simulink model "PEM_AFC"  (R2024a)
settings: Solver=FixedStepDiscrete  StartTime=0.0  StopTime=60  RelTol=1e-3  EnableMultiTasking=on
values from neighbouring files (symbols this model uses):
  alpha_bab = sqrt(Es / (SNR_linear * En_bab))    [Init_noise.m]
  alpha_imp = sqrt(Es / (SIR_linear * En_imp))    [Init_noise.m]
undefined symbols (not defined in the file or in its folder): a, delta, dfilt, dg, dk, framelength, g2, g4, mug, n_imp
libraries: dspobslib x6, dspvision x2, dspsrcs4 x2, dspswit3 x1, dspbuff3 x1, dspstat3 x1, dspsolvers x1, dspmathops x1
settings Model: Creator=Renato_Nakagawa  LastModifiedBy=tienc
settings SolverCC: AlgebraicLoopSolver=TrustRegion
settings DataIOCC: LimitDataPoints=on  SaveFormat=Array  ReturnWorkspaceOutputs=off
settings OptimizationCC: DefaultParameterBehavior=Inlined  EnhancedBackFolding=on  PassReuseOutputArgsAs=Individual arguments  ZeroExternalMemoryAtStartup=off  ZeroInternalMemoryAtStartup=off  OptimizeBlockOrder=speed  DifferentSizesBufferReuse=on  OptimizationCustomize=off  EfficientTunableParamExpr=on
settings DebuggingCC: UnderspecifiedInitializationDetection=Classic  MergeDetectMultiDrivingBlocksExec=none  SolverPrmCheckMsg=warning  ParameterTunabilityLossMsg=error  UnconnectedInputMsg=warning  UnconnectedOutputMsg=warning  UnconnectedLineMsg=warning  StateNameClashWarn=warning  SFUnexpectedBacktrackingDiag=warning  SFNoUnconditionalDefaultTransitionDiag=warning  SFExecutionAtInitializationDiag=none  ArithmeticOperatorsInVariantConditions=warning
settings HardwareCC: ProdBitPerPointer=32  ProdBitPerSizeT=32  ProdBitPerPtrDiffT=32  ProdLargestAtomicFloat=None  ProdIntDivRoundTo=Undefined  ProdEndianess=Unspecified  ProdWordSize=32  ProdHWDeviceType=32-bit Generic
settings ModelReferenceCC: PropagateSignalLabelsOutOfModel=off
settings SFSimCC: SimUseLocalCustomCode=off  MATLABDynamicMemAlloc=off  CustomCodeUndefinedFunction=UseInterfaceOnly
settings RTWCC: Description=Embedded Coder  SystemTargetFile=ert.tlc  GenCodeOnly=on  TemplateMakefile=ert_default_tmf  RTWUseLocalCustomCode=off  GPUComputeCapability=3.5
settings CodeAppCC: ForceParamTrailComments=on  IgnoreCustomStorageClasses=off  OperatorAnnotations=on  SimulinkDataObjDesc=on  SFDataObjDesc=on  InsertBlockDesc=on
settings ERTTargetCC: GenerateSampleERTMain=on  InlinedParameterPlacement=NonHierarchical  ERTCustomFileTemplate=example_file_process.tlc
settings ConfigComp: CovMetricSettings=dw  CovSaveCumulativeToWorkspaceVar=on  CovSaveSingleToWorkspaceVar=on  CovExternalEMLEnable=off  CovSFcnEnable=off

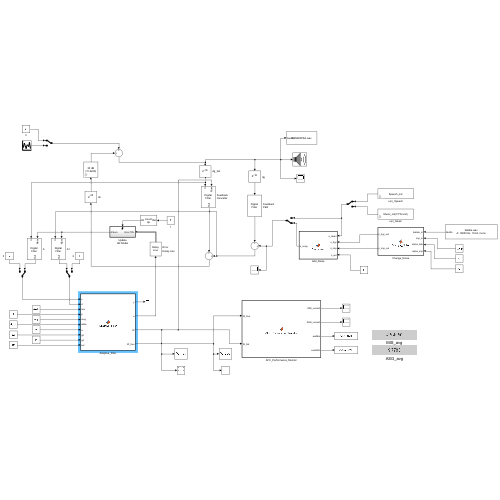
[thumbnail: Simulink's stored preview of the top-level diagram]
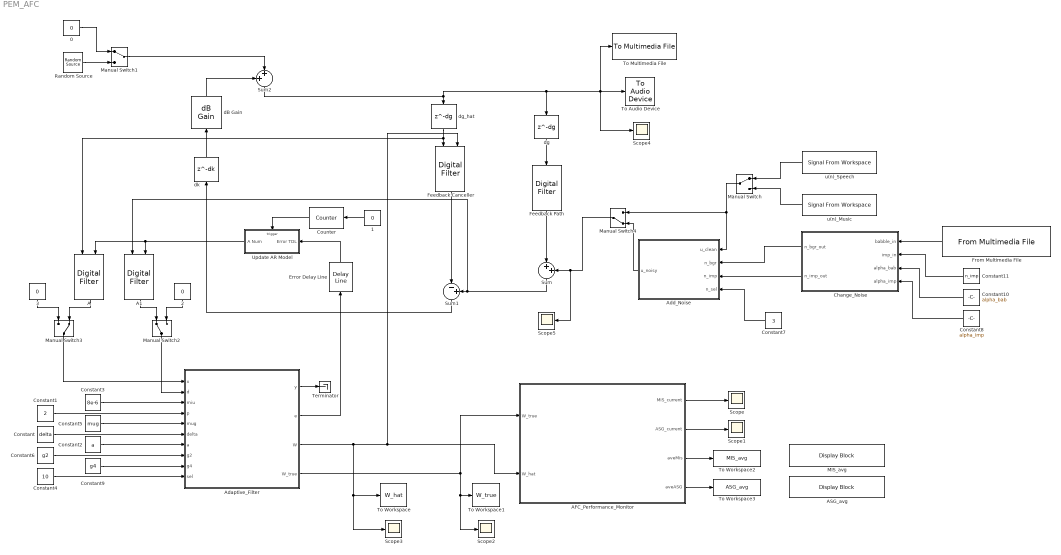
== system PEM_AFC ==
  {0..3} (4 alike) : Constant  Value=0
  A : dspobslib/Digital Filter  TypePopup=FIR (all zeros)  IIRFiltStruct=Direct form II transposed  AllPoleFiltStruct=Direct form  FIRFiltStruct=Direct form  CoeffSource=Input port(s)  NumCoeffs=g2  DenCoeffs=[1 0.1]  BiQuadCoeffs=[1 0.3 0.4 1 0.1 0.2]  LatticeCoeffs=[0.2 0.4]  denIgnore=on  FiltPerSampPopup=One filter per frame  IC=0  ICnum=0  ICden=0  roundingMode=Floor  overflowMode=off  ScaleValues=1  scaleValueFracLength=14  stageInFracLength=15  stageOutFracLength=15  FilterSource=Input port(s)  dfiltObjectName=dfilt.dffir([1 2 1])
  A1 : dspobslib/Digital Filter  TypePopup=FIR (all zeros)  IIRFiltStruct=Direct form II transposed  AllPoleFiltStruct=Direct form  FIRFiltStruct=Direct form  CoeffSource=Input port(s)  NumCoeffs=g2  DenCoeffs=[1 0.1]  BiQuadCoeffs=[1 0.3 0.4 1 0.1 0.2]  LatticeCoeffs=[0.2 0.4]  denIgnore=on  FiltPerSampPopup=One filter per frame  IC=0  ICnum=0  ICden=0  roundingMode=Floor  overflowMode=off  ScaleValues=1  scaleValueFracLength=14  stageInFracLength=15  stageOutFracLength=15  FilterSource=Input port(s)  dfiltObjectName=dfilt.dffir([1 2 1])
  AFC_Performance_Monitor : MATLAB Function  TreatAsAtomicUnit=on
  ASG_avg : DisplayBlock  LabelPosition=Hide  Transparency=1
  Adaptive_Filter : MATLAB Function  TreatAsAtomicUnit=on
  Add_Noise : MATLAB Function  TreatAsAtomicUnit=on
  Change_Noise : MATLAB Function  TreatAsAtomicUnit=on
  Constant : Constant  Value=delta
  Constant1 : Constant  Value=2
  Constant10 : Constant  Value=alpha_bab
  Constant11 : Constant  Value=n_imp
  Constant2 : Constant  Value=a
  Constant3 : Constant  Value=8e-6
  Constant4 : Constant  Value=10
  Constant5 : Constant  Value=mug
  Constant6 : Constant  Value=g2
  Constant7 : Constant  Value=3
  Constant8 : Constant  Value=alpha_imp
  Constant9 : Constant  Value=g4
  Counter : dspswit3/Counter  Direction=Up  CountEvent=Free running  CounterSize=User defined  MaxCount=framelength-1  InitialCount=0  Output=Hit  HitValue=framelength-1  ResetInput=on  SamplesPerFrame=1  Ts=1/16000  CntDtype=double  HitDtype=Boolean
  Error Delay Line : dspbuff3/Delay Line  siz=Nh  ic=0  directfeed=off  enable_output=off  hold_output=off  OutputFrames=on
  Feedback Canceller : dspobslib/Digital Filter  TypePopup=FIR (all zeros)  IIRFiltStruct=Direct form II transposed  AllPoleFiltStruct=Direct form  FIRFiltStruct=Direct form  CoeffSource=Input port(s)  NumCoeffs=g2  DenCoeffs=[1 0.1]  BiQuadCoeffs=[1 0.3 0.4 1 0.1 0.2]  LatticeCoeffs=[0.2 0.4]  denIgnore=on  FiltPerSampPopup=One filter per frame  IC=0  ICnum=0  ICden=0  roundingMode=Floor  overflowMode=off  ScaleValues=1  scaleValueFracLength=14  stageInFracLength=15  stageOutFracLength=15  FilterSource=Input port(s)  dfiltObjectName=dfilt.dffir([1 2 1])
  "Feedback Path " : dspobslib/Digital Filter  TypePopup=FIR (all zeros)  IIRFiltStruct=Direct form II transposed  AllPoleFiltStruct=Direct form  FIRFiltStruct=Direct form  CoeffSource=Specify via dialog  NumCoeffs=g2  DenCoeffs=[1 0.1]  BiQuadCoeffs=[1 0.3 0.4 1 0.1 0.2]  LatticeCoeffs=[0.2 0.4]  denIgnore=on  FiltPerSampPopup=One filter per frame  IC=0  ICnum=0  ICden=0  roundingMode=Floor  overflowMode=off  ScaleValues=1  scaleValueFracLength=14  stageInFracLength=15  stageOutFracLength=15  FilterSource=Specify via dialog  dfiltObjectName=dfilt.dffir([1 2 1])
  From Multimedia File : dspvision/From Multimedia File  inputFilename=C:\Documents\NCKH\IPAPSA for AFC using prefilter in HAs\Simulink\NOISEX-92\babble.wav  readRange=[1 Inf]  loop=on  numPlays=inf  outputStreams=Audio only  videoDataType=single  audioDataType=double  inheritSampleTime=off  userDefinedSampleTime=1/16000  noAudioOutput=off  isIntensityVideo=off  fourcc=RGB  colorVideoFormat=Separate color signals  outputEOF=off  dataOrg=Column-major  audioFrameSize=1  computeAudioFrameSize=off  outSamplingMode=Sample based
      settings: LibrarySourceBlock=audiosources/From Multimedia File
  MIS_avg : DisplayBlock  LabelPosition=Hide  Transparency=1
  Manual Switch : ManualSwitch
  Manual Switch1 : ManualSwitch
  Manual Switch2 : ManualSwitch
  Manual Switch3 : ManualSwitch  CurrentSetting=0
  Manual Switch4 : ManualSwitch  CurrentSetting=0
  Random Source : dspobslib/Random Source  SrcType=Gaussian  NormMethod=Ziggurat  CltLength=12  MinVal=0  MaxVal=1  MeanVal=0  VarVal=var  RepMode=Not repeatable  rawSeed=1  IsInherit=off  SampMode=Discrete  SampTime=1/16000  SampFrame=1  DataType=Double  OutComplex=Real  OutputFrames=on
  Scope{,1..5} (6 alike) : Scope
  Sum : Sum  Inputs=|++
  Sum1 : Sum  Inputs=|-+
  Sum2 : Sum  Inputs=++|
  Terminator : Terminator
  To Audio Device : dspobslib/To Audio Device  deviceName=Default  inheritSampleRate=on  sampleRate=44100  deviceDatatype=Determine from input data type  autoBufferSize=on  bufferSize=4096  queueDuration=1.0  defaultOutputChannelMapping=on  outputChannelMapping=1  outputNumUnderrunSamples=off
  To Multimedia File : dspvision/To Multimedia File  outputFilename=BSMIPAPSA.wav  streamSelection=Audio only  videoCompressor=None (uncompressed)  audioCompressor=None (uncompressed)  imagePorts=One multidimensional signal  fileType=WAV  audioDatatype=16-bit integer  fourcc=RGB  audioBitRate=128  audioQuality=75  videoQuality=75  mj2000CompFactor=10
      settings: LibrarySourceBlock=audiosinks/To Multimedia File
  To Workspace : ToWorkspace  VariableName=W_hat  SampleTime=-1
      settings: Save2DSignal=2-D array (concatenate along first dimension)
  To Workspace1 : ToWorkspace  VariableName=W_true  SampleTime=-1
      settings: Save2DSignal=2-D array (concatenate along first dimension)
  To Workspace2 : ToWorkspace  VariableName=MIS_avg  SampleTime=-1
      settings: Save2DSignal=2-D array (concatenate along first dimension)
  To Workspace3 : ToWorkspace  VariableName=ASG_avg  SampleTime=-1
      settings: Save2DSignal=2-D array (concatenate along first dimension)
  Update AR Model : Subsystem  TreatAsAtomicUnit=on
  dB Gain : dspmathops/dB Gain  dB=K_dB  intype=Amplitude
  dg : Delay  DelayLength=dg  InitialCondition=0
  dg_hat : Delay  DelayLength=dg  InitialCondition=0
  dk : Delay  DelayLength=dk  InitialCondition=0
  u(n)_Music : dspsrcs4/Signal From Workspace  X=Music_m4(15*fs:end)  Ts=1/16000  nsamps=1  OutputAfterFinalValue=Setting to zero  ignoreOrWarnInputAndFrameLengths=off  OutputFrames=on
  u(n)_Speech : dspsrcs4/Signal From Workspace  X=Speech_m2  Ts=1/16000  nsamps=1  OutputAfterFinalValue=Setting to zero  ignoreOrWarnInputAndFrameLengths=off  OutputFrames=on
  wires:
  dk/1 -> dB Gain/1
  dg_hat/1 -> Feedback Canceller/1, A/1
  Sum1/1 -> dk/1
  dB Gain/1 -> Sum2/1
  Error Delay Line/1 -> Update AR Model/1(Error TDL)
  Counter/1 -> Update AR Model/Trigger
  Sum/1 -> Sum1/2, A1/1
  Update AR Model/1(A Num) -> A1/2, A/2
  u(n)_Speech/1 -> Manual Switch/1
  u(n)_Music/1 -> Manual Switch/2
  Manual Switch1/1 -> Sum2/2
  Random Source/1 -> Manual Switch1/2
  0/1 -> Manual Switch1/1
  1/1 -> Counter/1
  Constant5/1 -> Adaptive_Filter/5(mug)
  Adaptive_Filter/1(y) -> Terminator/1
  Adaptive_Filter/2(e) -> Error Delay Line/1
  Constant/1 -> Adaptive_Filter/6(delta)
  Constant1/1 -> Adaptive_Filter/4(p)
  Constant2/1 -> Adaptive_Filter/7(a)
  Constant4/1 -> Adaptive_Filter/10(sel)
  Constant3/1 -> Adaptive_Filter/3(miu)
  3/1 -> Manual Switch3/1
  A/1 -> Manual Switch3/2
  A1/1 -> Manual Switch2/1
  2/1 -> Manual Switch2/2
  Manual Switch3/1 -> Adaptive_Filter/1(x)
  Manual Switch2/1 -> Adaptive_Filter/2(d)
  AFC_Performance_Monitor/1(MIS_current) -> Scope/1
  Adaptive_Filter/3(W) -> Feedback Canceller/2, AFC_Performance_Monitor/2(W_hat), To Workspace/1, Scope3/1
  Sum2/1 -> To Multimedia File/1, Scope4/1, To Audio Device/1, dg/1, dg_hat/1
  Feedback Canceller/1 -> Sum1/1
  AFC_Performance_Monitor/3(aveMis) -> To Workspace2/1
  AFC_Performance_Monitor/4(aveASG) -> To Workspace3/1
  AFC_Performance_Monitor/2(ASG_current) -> Scope1/1
  dg/1 -> "Feedback Path "/1
  "Feedback Path "/1 -> Sum/1
  Constant6/1 -> Adaptive_Filter/8(g2)
  Constant9/1 -> Adaptive_Filter/9(g4)
  Adaptive_Filter/4(W_true) -> AFC_Performance_Monitor/1(W_true), Scope2/1, To Workspace1/1
  Constant7/1 -> Add_Noise/4(n_sel)
  Manual Switch/1 -> Manual Switch4/1, Add_Noise/1(u_clean)
  From Multimedia File/1 -> Change_Noise/1(babble_in)
  Constant10/1 -> Change_Noise/3(alpha_bab)
  Constant8/1 -> Change_Noise/4(alpha_imp)
  Change_Noise/1(n_bgr_out) -> Add_Noise/2(n_bgr)
  Change_Noise/2(n_imp_out) -> Add_Noise/3(n_imp)
  Constant11/1 -> Change_Noise/2(imp_in)
  Manual Switch4/1 -> Scope5/1, Sum/2
  Add_Noise/1(u_noisy) -> Manual Switch4/2

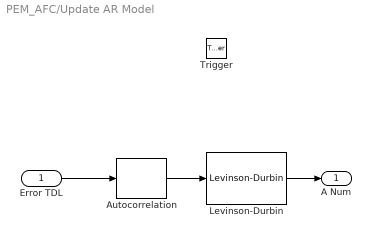
== system PEM_AFC/Update AR Model ==
  Error TDL : Inport
  Trigger : TriggerPort  VariantControl=(inherit)  ZeroCross=off
  Autocorrelation : dspstat3/Autocorrelation  AllPositiveLags=on  maxlag=1  bias=Unbiased  domain=Time  roundingMode=Floor  overflowMode=off  outputDataTypeStr=Inherit: Same as accumulator  outputMin=[]  outputMax=[]  outputLastDataTypeStr=Inherit: Same as accumulator
  Levinson-Durbin : dspsolvers/Levinson-Durbin  coeffOutFcn=OBSOLETE  coeffOutFcnActive=A  outP=off  zeroInpHandling=on  roundingMode=Floor  overflowMode=off  prodOutputMode=User-defined  prodOutputWordLength=32  prodOutputFracLength=30  prodOutputDataTypeStr=fixdt(1,32,30)  prodOutputLastDataTypeStr=fixdt(1,32,30)  accumMode=User-defined  accumWordLength=32  accumFracLength=30  accumDataTypeStr=fixdt(1,32,30)  accumLastDataTypeStr=fixdt(1,32,30)  firstCoeffMode=Binary point scaling  firstCoeffWordLength=16  firstCoeffFracLength=15  firstCoeffDataTypeStr=fixdt(1,16,15)  firstCoeffMin=[]  firstCoeffMax=[]  firstCoeffLastDataTypeStr=fixdt(1,16,15)  secondCoeffMode=Binary point scaling  secondCoeffWordLength=16  secondCoeffFracLength=15  secondCoeffDataTypeStr=fixdt(1,16,15)  secondCoeffMin=[]  secondCoeffMax=[]  secondCoeffLastDataTypeStr=fixdt(1,16,15)  outputMin=[]  outputMax=[]
      settings: allowOverrides=off
  A Num : Outport
  wires:
  Autocorrelation/1 -> Levinson-Durbin/1
  Error TDL/1 -> Autocorrelation/1
  Levinson-Durbin/1 -> A Num/1

== matlab function PEM_AFC/AFC_Performance_Monitor ==
  data: W_true input; W_hat input; MIS_current output; ASG_current output; aveMis output; aveASG output
function [MIS_current, ASG_current, aveMis, aveASG] = AFC_Performance_Monitor(W_true, W_hat)
% AFC_Performance_Monitor
% Tính MIS (Misalignment) và ASG (Added Stable Gain) theo từng mẫu để
% xuất trực tiếp sang Scope trong Simulink. Đồng thời duy trì giá trị
% trung bình (running average) của MIS và ASG trong suốt phiên mô phỏng.
%
% INPUTS:
%   W_true : vector hệ số feedback path thật (kích thước Lx1 hoặc 1xL)
%   W_hat  : vector hệ số ước lượng (kích thước Lx1 hoặc 1xL)
%
% OUTPUTS:
%   MIS_current : giá trị MIS hiện thời (dB)
%   ASG_current : giá trị ASG hiện thời (dB)
%   aveMis      : trung bình MIS tính đến thời điểm hiện tại (dB)
%   aveASG      : trung bình ASG tính đến thời điểm hiện tại (dB)

% Chuẩn hóa kích thước vector cột
g_current = W_true(:);
g_hat_current = W_hat(:);

% Độ dài bộ lọc và Nfreq đồng bộ theo MIS_cal.m / PEM_TDfeedback_Modified_simulink.m
filter_length = length(g_current);
if filter_length == 0
    MIS_current = 0; ASG_current = 0; aveMis = 0; aveASG = 0; return; %#ok<*NASGU>
end
Nfreq = filter_length;

% Biến persistent cho trung bình cộng dồn
persistent sumMIS sumASG nSamples
if isempty(nSamples)
    sumMIS = 0;
    sumASG = 0;
    nSamples = 0;
end

% Tiền xử lý đồng bộ MIS_cal.m / PEM_TDfeedback_Modified_simulink.m
% - Remove DC cho đường thật
% - Chèn trễ d_fb cho cả thật và ước lượng
d_fb = 16; % phải trùng với mô phỏng
g_true_nodc = g_current - mean(g_current);
g_true_delayed = [zeros(d_fb,1); g_true_nodc; 0];
g_hat_delayed  = [zeros(d_fb,1); g_hat_current];

% Phổ tần số của hệ số thật và ước lượng
G_freq = fft(g_true_delayed, Nfreq);
G_hat_freq = fft(g_hat_delayed, Nfreq);

% Sai số ước lượng ở miền tần số (nửa dải tần)
half_idx = 1:ceil(Nfreq/2);
G_tilde = G_freq(half_idx) - G_hat_freq(half_idx);

% MIS hiện thời (đồng bộ công thức)
den_norm = norm(G_freq(half_idx));
% Thêm eps nhỏ để tránh NaN trong mô phỏng số mà không thay đổi định nghĩa
MIS_current = 20*log10(norm(G_tilde)/(den_norm + eps));

% MSG và ASG hiện thời (đồng bộ phạm vi tần số của ASG: 1:Nfreq/2+1)
G_tilde_abs = abs(G_tilde);
MSG_current = 20*log10(min(1./(G_tilde_abs + eps)));
G_freq_abs = abs(G_freq(1:(Nfreq/2+1)));
ASG_current = MSG_current - 20*log10(min(1./(G_freq_abs + eps)));

% Cập nhật trung bình cộng dồn
nSamples = nSamples + 1;
sumMIS = sumMIS + MIS_current;
sumASG = sumASG + ASG_current;
aveMis = sumMIS / nSamples;
aveASG = sumASG / nSamples;

end

== matlab function PEM_AFC/Adaptive_Filter ==
  data: x input; d input; miu input; p input; y output; mug input; e output; W output; delta input; a input; g2 input; g4 input; sel input; W_true output
function [y, e, W, W_true] = Adaptive_Filter(x, d, miu, p, mug, delta, a, g2, g4, sel)
    % --- KHAI BÁO HẰNG SỐ CỐ ĐỊNH ---
    FILTER_ORDER = 64;   
    MAX_P = 10;
    AR_ORDER = 20;
    FRAMELENGTH = 160;
    
    % --- KIỂM TRA ĐẦU VÀO ---
    assert(p <= MAX_P);          
    assert(p >= 1);
    
    % Khởi tạo outputs
    y = 0.0;
    e = 0.0;
    W = zeros(FILTER_ORDER, 1);
    W_true = zeros(FILTER_ORDER, 1);

    % Persistent variables
    persistent AF AR;
    persistent sample_counter feedback_path_changed;
    persistent change_sample current_feedback_path;

    %% --- KHỞI TẠO (INITIALIZATION) ---
    if isempty(AF)
        % Khởi tạo AF structure
        AF.gTD = zeros(FILTER_ORDER, 1);
        AF.N = FILTER_ORDER;
        AF.mu = miu;
        AF.delta = delta;
        AF.TDLLs = zeros(FILTER_ORDER, 1);
        AF.TDLLswh = zeros(FILTER_ORDER, 1);
        
        % Khởi tạo mảng cho APA (Kích thước tĩnh MAX_P)
        AF.P = p; 
        AF.TDLLswh_d = zeros(FILTER_ORDER + MAX_P - 1, 1); 
        AF.TDLMicwh = zeros(MAX_P, 1);     
        AF.Lswh_ap = zeros(FILTER_ORDER, MAX_P); 
        
        AF.delta_IPAPA = 0;
        AF.mu1 = 0.5 * mug;
        AF.mu2 = 0.1 * mug;
        
        % Khởi tạo cho PEM-IPAPSA / PEM-MIPAPSA / PEM-BSMIPAPSA
        AF.Q_tilde_prev = zeros(FILTER_ORDER, MAX_P - 1);
        
        % Khởi tạo AR structure
        AR.N = AR_ORDER;
        AR.w = [1; zeros(AR_ORDER-1, 1)];
        AR.framelength = FRAMELENGTH;
        AR.frameindex = 0;
        AR.TDLMicdelay = zeros(FRAMELENGTH+1, 1);
        AR.TDLLsdelay = zeros(FRAMELENGTH+1, 1);
        % Đây là biến gây lỗi lúc nãy, nó đã được khai báo ở đây là TDLMicwh
        AR.TDLMicwh = zeros(AR_ORDER, 1); 
        AR.TDLLswh = zeros(AR_ORDER, 1);
        AR.frame = zeros(FRAMELENGTH, 1);
        
        % Feedback path logic
        sample_counter = 0;
        feedback_path_changed = false;
        change_sample = 480000;
        current_feedback_path = 1;
    end

    %% --- XỬ LÝ CHÍNH (MAIN PROCESSING) ---
    % Chuẩn hóa input
    if ~isscalar(x), x = x(1); end
    if ~isscalar(d), d = d(1); end

    % Feedback path switching
    sample_counter = sample_counter + 1;
    if sample_counter >= 960000
        sample_counter = 0;
        feedback_path_changed = false;
        current_feedback_path = 1;
    end
    if sample_counter >= change_sample && ~feedback_path_changed
        feedback_path_changed = true;
        current_feedback_path = 2;
    end

    AF.mu = miu;
    
    % 1. Cập nhật TDLLs
    AF.TDLLs = [x; AF.TDLLs(1:end-1,1)];
    
    % 2. Tính error signal
    e = d - AF.gTD' * AF.TDLLs;
    
    % 3. Clipping
    e = 2*tanh(0.5*e);
    
    % 4, 5. Delay & Filter signals
    [Micdelay, AR.TDLMicdelay] = delay_sample_inline(d, AR.framelength, AR.TDLMicdelay);
    [Lsdelay, AR.TDLLsdelay] = delay_sample_inline(x, AR.framelength, AR.TDLLsdelay);
    
    % [ĐÃ SỬA LỖI TẠI ĐÂY] Dùng đúng tên biến AR.TDLMicwh
    [Micwh, AR.TDLMicwh] = filter_sample_inline(Micdelay, AR.w, AR.TDLMicwh);
    [Lswh, AR.TDLLswh] = filter_sample_inline(Lsdelay, AR.w, AR.TDLLswh);

    % 6. Update AR-model
    AR.frame(2:AR.framelength) = AR.frame(1:AR.framelength-1);
    AR.frame(1) = e;
    
    % Levinson Logic
    if and(AR.frameindex == AR.framelength-1, AR.N-1 > 0)
        R = zeros(AR.N, 1);
        for j = 1:AR.N
            frame_segment = AR.frame(j:end);
            pad_zeros = zeros(j-1, 1);
            vec_mult = [frame_segment; pad_zeros];
            R(j,1) = (AR.frame' * vec_mult) / AR.framelength;
        end
        [ar_coeffs, ~] = levinson(R, AR.N-1);
        AR.w(1:length(ar_coeffs)) = ar_coeffs';
        AR.w(length(ar_coeffs)+1:end) = 0;
    end
    AR.frameindex = AR.frameindex + 1;
    if AR.frameindex == AR.framelength
        AR.frameindex = 0;
    end

    % 7. Update TDLLswh
    AF.TDLLswh = [Lswh; AF.TDLLswh(1:end-1,1)];
    
    % 8. Calculate ep
    ep = Micwh - AF.gTD' * AF.TDLLswh;

    %% --- XỬ LÝ APA/IPAPA (Static Memory) ---
    AF.TDLMicwh = [Micwh; AF.TDLMicwh(1:end-1, 1)];
    AF.TDLLswh_d = [Lswh; AF.TDLLswh_d(1:end-1, 1)];
    
    for i = 1:p 
        vec_start = i;
        vec_end = i + FILTER_ORDER - 1;
        if vec_end <= length(AF.TDLLswh_d)
            col_vec = AF.TDLLswh_d(vec_start : vec_end);
        else
            col_vec = zeros(FILTER_ORDER, 1);
            avail = length(AF.TDLLswh_d) - vec_start + 1;
            col_vec(1:avail) = AF.TDLLswh_d(vec_start:end);
        end
        AF.Lswh_ap(:, i) = col_vec; 
    end
    
    Lswh_ap_active = AF.Lswh_ap(:, 1:p); 
    TDLMicwh_active = AF.TDLMicwh(1:p);
    ewh_p = TDLMicwh_active - Lswh_ap_active' * AF.gTD;

    %% --- THUẬT TOÁN THÍCH NGHI ---
    if sel == 1      % NLMS
        AF.gTD = AF.gTD + (AF.mu / (norm(AF.TDLLswh)^2 + AF.delta)) * AF.TDLLswh .* ep;
        
    elseif sel == 2  % IPNLMS
        aa = a;
        kd = (1 - aa) / (2 * length(AF.gTD)) + (1 + aa) * abs(AF.gTD) / (AF.delta + 2 * sum(abs(AF.gTD)));
        Kd = diag(kd);
        denom = AF.TDLLswh' * Kd * AF.TDLLswh + AF.delta * (1 - aa) / (2 * length(AF.gTD));
        AF.gTD = AF.gTD + (AF.mu / denom) * Kd * AF.TDLLswh .* ep;
        
    elseif sel == 3  % HNLMS
        hv = e;
        e_clipped = 2*tanh(0.5*e);
        aaa = (abs(hv - e_clipped) < 0.15);
        if ~isfield(AF, 'mu1'), AF.mu1 = 0.1 * mug; end
        if ~isfield(AF, 'mu2'), AF.mu2 = 20 * mug; end
        PEMSC_NLMS_term = AF.TDLLswh .* ep / (norm(AF.TDLLswh)^2 + AF.delta);
        NLMS_term = AF.TDLLs .* e / (norm(AF.TDLLs)^2 + AF.delta);
        AF.gTD = AF.gTD + aaa * AF.mu1 * PEMSC_NLMS_term + (1 - aaa) * AF.mu2 * NLMS_term;
        
    elseif sel == 4  % APA
        AtA = Lswh_ap_active' * Lswh_ap_active;
        A_mat = AF.delta * eye(p) + AtA;
        rc = rcond(A_mat);
        if ~isfinite(rc) || rc < 1e-10
            A_mat = A_mat + (max(AF.delta, 1e-6) * 10) * eye(p);
        end
        update = Lswh_ap_active * (A_mat \ ewh_p);
        AF.gTD = AF.gTD + AF.mu * update;
        
    elseif sel == 5  % IPAPA
        aa = a;
        AF.delta_IPAPA = AF.delta * (1 - aa) / (2 * length(AF.gTD));
        kd = (1 - aa) / (2 * length(AF.gTD)) + (1 + aa) * abs(AF.gTD) / (AF.delta + 2 * sum(abs(AF.gTD)));
        Kd = diag(kd);
        AtKA = Lswh_ap_active' * Kd * Lswh_ap_active;
        B_mat = AtKA + AF.delta_IPAPA * eye(p);
        rb = rcond(B_mat);
        if ~isfinite(rb) || rb < 1e-10
            B_mat = B_mat + (max(AF.delta_IPAPA, 1e-6) * 10) * eye(p);
        end
        update = Kd * Lswh_ap_active * (B_mat \ ewh_p);
        AF.gTD = AF.gTD + AF.mu * update;
        
    elseif sel == 6  % PEM-IPAPSA (Improved Proportionate APSA)
        % Tham số proportionate
        aa = a;  % beta trong bài báo
        xi = AF.delta;  % xi = delta = 1e-6
        eps_val = (1 - aa) / (2 * FILTER_ORDER) * AF.delta;  % epsilon
        
        % 1. Tính proportionate vector b_k(n) - eq.(16)
        b = (1 - aa) / (2 * FILTER_ORDER) + ...
            (1 + aa) * abs(AF.gTD) / (sum(abs(AF.gTD)) + xi);
        B = diag(b);
        
        % 2. Tính u_{p,gs}(n) = B(n) * U_p(n) * sgn(e_p(n)) - eq.(15)
        u_pgs = B * Lswh_ap_active * sign(ewh_p);
        
        % 3. Cập nhật trọng số - eq.(18)
        denom = sqrt(u_pgs' * u_pgs + eps_val);
        AF.gTD = AF.gTD + AF.mu * u_pgs / denom;
        
    elseif sel == 7  % PEM-MIPAPSA (Memory Improved PAPSA)
        % Tham số proportionate
        aa = a;
        xi = AF.delta;
        eps_val = (1 - aa) / (2 * FILTER_ORDER) * AF.delta;
        
        % 1. Tính proportionate vector b(n) - eq.(16)
        b = (1 - aa) / (2 * FILTER_ORDER) + ...
            (1 + aa) * abs(AF.gTD) / (sum(abs(AF.gTD)) + xi);
        
        % 2. Xây dựng Q_tilde(n) với memory - eq.(19)-(20)
        %    Cột đầu tiên: b(n) .* u_p(n) (hiện tại)
        %    Các cột còn lại: Q_tilde_prev (từ step trước)
        current_col = b .* Lswh_ap_active(:, 1);  % b(n) ⊙ u_p(n)
        
        if p >= 2
            Q_tilde = zeros(FILTER_ORDER, p);
            Q_tilde(:, 1) = current_col;
            cols_from_prev = min(p - 1, size(AF.Q_tilde_prev, 2));
            Q_tilde(:, 2:1+cols_from_prev) = AF.Q_tilde_prev(:, 1:cols_from_prev);
        else
            Q_tilde = current_col;
        end
        
        % 3. Tính u_tilde_{p,gs}(n) = Q_tilde(n) * sgn(e_p(n)) - eq.(20)
        u_tilde_pgs = Q_tilde * sign(ewh_p);
        
        % 4. Cập nhật trọng số - eq.(21)
        denom = sqrt(u_tilde_pgs' * u_tilde_pgs + eps_val);
        AF.gTD = AF.gTD + AF.mu * u_tilde_pgs / denom;
        
        % 5. Lưu Q_tilde_prev cho step tiếp theo (shift columns)
        if p >= 2
            AF.Q_tilde_prev(:, 2:end) = AF.Q_tilde_prev(:, 1:end-1);
            AF.Q_tilde_prev(:, 1) = current_col;
        end
        
    elseif sel == 8  % PEM-BSMIPAPSA (Block-Sparse Memory IPAPSA)
        % Tham số proportionate
        aa = a;
        xi = AF.delta;
        eps_val = (1 - aa) / (2 * FILTER_ORDER) * AF.delta;
        
        % 1. Xác định số blocks M và chiều dài block N
        M_bs = 8;  
        N_bs = FILTER_ORDER / M_bs;
        
        % 2. Tính block-sparse proportionate vector - eq.(24)
        b_hat = zeros(FILTER_ORDER, 1);
        block_norms = zeros(M_bs, 1);
        for blk = 1:M_bs
            idx_start = (blk - 1) * N_bs + 1;
            idx_end = blk * N_bs;
            block_norms(blk) = norm(AF.gTD(idx_start:idx_end), 2);
        end
        sum_block_norms = sum(block_norms);
        
        for blk = 1:M_bs
            idx_start = (blk - 1) * N_bs + 1;
            idx_end = blk * N_bs;
            b_hat_k = (1 - aa) / (2 * FILTER_ORDER) + ...
                      (1 + aa) * block_norms(blk) / (2 * M_bs * sum_block_norms + xi);
            b_hat(idx_start:idx_end) = b_hat_k;
        end
        
        % 3. Xây dựng Q_hat(n) với memory - eq.(23),(25)
        current_col = b_hat .* Lswh_ap_active(:, 1);  % b_hat(n) ⊙ u_p(n)
        
        if p >= 2
            Q_hat = zeros(FILTER_ORDER, p);
            Q_hat(:, 1) = current_col;
            cols_from_prev = min(p - 1, size(AF.Q_tilde_prev, 2));
            Q_hat(:, 2:1+cols_from_prev) = AF.Q_tilde_prev(:, 1:cols_from_prev);
        else
            Q_hat = current_col;
        end
        
        % 4. Tính u_hat_{p,gs}(n) = Q_hat(n) * sgn(e_p(n))
        u_hat_pgs = Q_hat * sign(ewh_p);
        
        % 5. Cập nhật trọng số - eq.(25)
        denom = sqrt(u_hat_pgs' * u_hat_pgs + eps_val);
        AF.gTD = AF.gTD + AF.mu * u_hat_pgs / denom;
        
        % 6. Lưu Q_tilde_prev cho step tiếp theo (dùng chung buffer)
        if p >= 2
            AF.Q_tilde_prev(:, 2:end) = AF.Q_tilde_prev(:, 1:end-1);
            AF.Q_tilde_prev(:, 1) = current_col;
        end
    end

    % Output
    % FIX CODER ERROR: Ép cố định kích thước của W_true là FILTER_ORDER x 1
    % Tránh việc Simulink hiểu nhầm W_true bị đổi kích thước (variable-size) do g2/g4
    W_true = zeros(FILTER_ORDER, 1);
    if current_feedback_path == 1
        len_g2 = min(length(g2), FILTER_ORDER);
        W_true(1:len_g2) = g2(1:len_g2);
    else
        len_g4 = min(length(g4), FILTER_ORDER);
        W_true(1:len_g4) = g4(1:len_g4);
    end
    W = AF.gTD;
end

%% Helper Functions
function [output, delayline_out] = delay_sample_inline(x, delay, delayline_in)
    delayline_out = [x; delayline_in(1:end-1,:)];
    output = delayline_out(delay+1,:);
end

function [output, delayline_out] = filter_sample_inline(x, w, delayline_in)
    delayline_out = [x; delayline_in(1:end-1,:)];
    output = delayline_out' * w;
end

== matlab function PEM_AFC/Add_Noise ==
  data: u_clean input; u_noisy output; n_bgr input; n_imp input; n_sel input
function u_noisy = Add_noise(u_clean, n_bgr, n_imp, n_sel)
% ADD_NOISE - Simulink MATLAB Function Block
% Thêm nhiễu nền và nhiễu xung vào tín hiệu speech/music sạch.
%
% Tất cả nhiễu đã được tiền xử lý (resample + scale theo SNR/SIR)
% trong script Init_noise.m và đưa vào qua "From Workspace" block.
%
% INPUTS:
%   u_clean : Mẫu tín hiệu sạch (speech hoặc music), scalar
%             Đến từ nguồn speech/music có sẵn trong Simulink
%   n_bgr   : Mẫu nhiễu nền đã scale (babble/factory/white...), scalar
%             Đến từ "From Workspace" block (ts_bgr_babble)
%   n_imp   : Mẫu nhiễu xung đã scale (Bernoulli-Gaussian), scalar
%             Đến từ "From Workspace" block (ts_n_imp)
%   n_sel   : Chọn chế độ thêm nhiễu, scalar
%             0 = không thêm nhiễu (giữ nguyên tín hiệu sạch)
%             1 = chỉ thêm nhiễu nền (background noise)
%             2 = chỉ thêm nhiễu xung (impulsive noise)
%             3 = thêm cả nhiễu nền + nhiễu xung (giống Hệ thống A)
%
% OUTPUT:
%   u_noisy : Mẫu tín hiệu đã thêm nhiễu, scalar

    if n_sel == 0
        % Không thêm nhiễu
        u_noisy = u_clean;
    elseif n_sel == 1
        % Chỉ thêm nhiễu nền (babble/factory/white...)
        u_noisy = u_clean + n_bgr;
    elseif n_sel == 2
        % Chỉ thêm nhiễu xung (impulsive)
        u_noisy = u_clean + n_imp;
    else
        % n_sel == 3 hoặc khác: Thêm cả hai (giống Hệ thống A)
        % Tương ứng: u = u_bab + scaled_imp trong Hệ thống A
        u_noisy = u_clean + n_bgr + n_imp;
    end

end

== matlab function PEM_AFC/Change_Noise ==
  data: babble_in input; imp_in input; alpha_bab input; n_bgr_out output; alpha_imp input; n_imp_out output
function [n_bgr_out, n_imp_out] = Change_Noise(babble_in, imp_in, alpha_bab, alpha_imp)
% =========================================================================
% CHANGE_NOISE - Simulink MATLAB Function Block
%
% Scale nhiễu bằng hệ số alpha CỐ ĐỊNH (đã tính sẵn trong workspace
% bởi Init_noise.m), giống hệt hàm add_noise.m của Hệ thống A.
%
% INPUTS:
%   babble_in  : Nhiễu babble từ "From Multimedia File" (scalar, đã resample)
%   imp_in     : Nhiễu xung - TOÀN BỘ vector n_imp từ workspace (960000x1)
%   alpha_bab  : Hệ số scale babble (Constant block, tính từ Init_noise.m)
%   alpha_imp  : Hệ số scale impulsive (Constant block, tính từ Init_noise.m)
%
% OUTPUTS:
%   n_bgr_out  : Nhiễu nền đã scale (scalar) → đưa vào Add_noise
%   n_imp_out  : Nhiễu xung đã scale (scalar) → đưa vào Add_noise
% =========================================================================

    % Biến đếm để trích từng mẫu từ vector imp_in
    persistent idx
    if isempty(idx)
        idx = 1;
    end

    % --- TRÍCH MẪU NHIỄU XUNG ---
    if length(imp_in) > 1
        % imp_in là vector đầy đủ từ workspace
        if idx <= length(imp_in)
            current_imp = imp_in(idx);
        else
            current_imp = 0;
        end
        idx = idx + 1;
    else
        % imp_in đã là scalar
        current_imp = imp_in;
    end

    % --- SCALE NHIỄU (giống hệt add_noise.m: scaledNoise = alpha * n) ---
    n_bgr_out = alpha_bab * babble_in;
    n_imp_out = alpha_imp * current_imp;

end
